simulink model "Practica1a__SemModSimulSist_Simulink"  (R2025b)
settings: Solver=VariableStepAuto  StartTime=0.0  StopTime=10.0  RelTol=1e-3
PreLoadFcn:
  | Ip = 0.0079;
  | Mc = 0.7031;
  | Lp = 0.3302;
  | Mp = 0.23;
  | Fc = 0;
  | Beq = 4.3;
  | g = 9.81;
  | Bp = 0.0024;
  | 
  | A = (Ip + Mp*(Lp^2))*Fc;
  | B = (Mp^2)*(Lp^2)*g;
  | C = (Ip + Mp*(Lp^2))*Beq;
  | D = Ip*Mp*Lp + (Mp^2)*(Lp^3); % Se cambio signo
  | E = Mp*Lp*Bp;
  | F = (Mc + Mp)*Mp*g*Lp;
  | G = (Mc + Mp)*Bp;
  | H = Fc*Mp*Lp;
  | K = (Mp^2)*(Lp^2);
  | M = Beq*Mp*Lp;
  | N = (Mc + Mp)*Ip + Mc*Mp*(Lp^2);
  | P = (Mp^2)*(Lp^2);
InitFcn:
  | Ip = 0.0079;
  | Mc = 0.7031;
  | Lp = 0.3302;
  | Mp = 0.23;
  | Fc = 0;
  | Beq = 4.3;
  | g = 9.81;
  | Bp = 0.0024;
  | 
  | 
  | A = (Ip + Mp*(Lp^2))*Fc;
  | 
  | B = (Mp^2)*(Lp^2)*g;
  | 
  | C = (Ip + Mp*(Lp^2))*Beq;
  | 
  | D = Ip*Mp*Lp + (Mp^2)*(Lp^3); % Se cambio signo
  | 
  | E = Mp*Lp*Bp;
  | 
  | F = (Mc + Mp)*Mp*g*Lp;
  | 
  | G = (Mc + Mp)*Bp;
  | 
  | H = Fc*Mp*Lp;
  | 
  | K = (Mp^2)*(Lp^2);
  | 
  | M = Beq*Mp*Lp;
  | 
  | N = (Mc + Mp)*Ip + Mc*Mp*(Lp^2);
  | 
  | P = (Mp^2)*(Lp^2);
undefined symbols (not defined in the file): magnitude
settings Model: Creator=jlsot  LastModifiedBy=jlsot

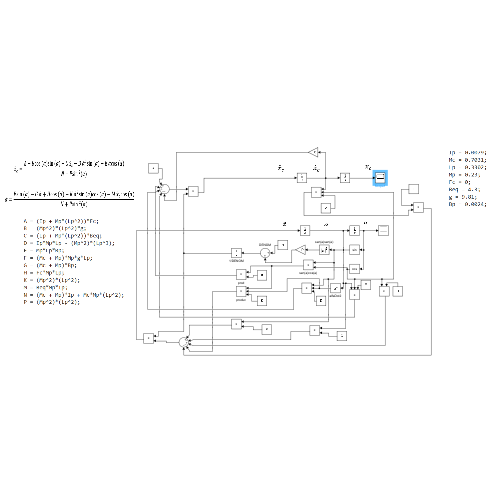
[thumbnail: Simulink's stored preview of the top-level diagram]
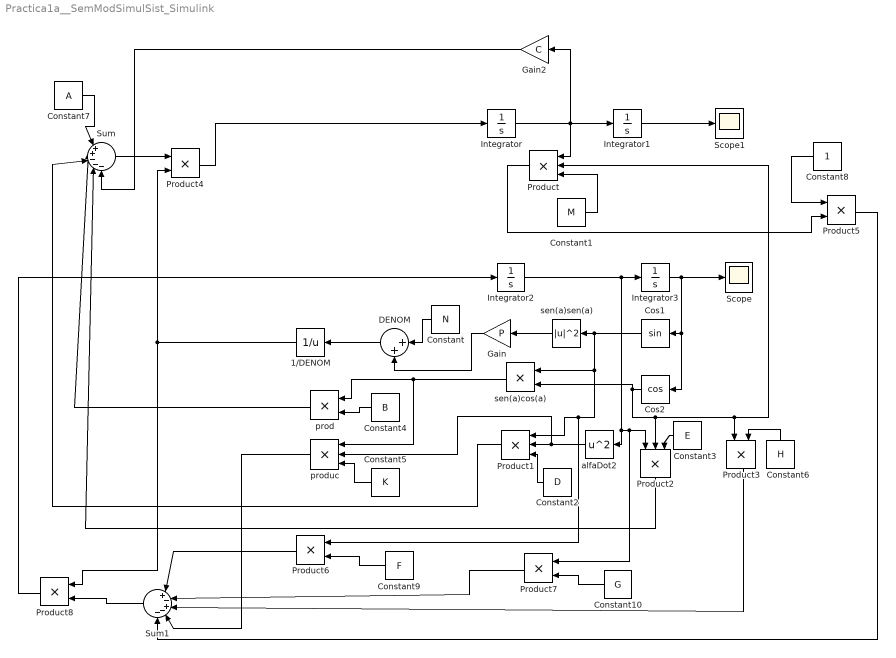
== system Practica1a__SemModSimulSist_Simulink ==
  1/DENOM : Math  Operator=reciprocal  SignedPower=on
  Constant : Constant  Value=N
  Constant1 : Constant  Value=M
  Constant10 : Constant  Value=G
  Constant2 : Constant  Value=D
  Constant3 : Constant  Value=E
  Constant4 : Constant  Value=B
  Constant5 : Constant  Value=K
  Constant6 : Constant  Value=H
  Constant7 : Constant  Value=A
  Constant8 : Constant
  Constant9 : Constant  Value=F
  Cos1 : Trigonometry
  Cos2 : Trigonometry  Operator=cos
  DENOM : Sum  Inputs=|++
  Gain : Gain  Gain=P
  Gain2 : Gain  Gain=C
  Integrator : Integrator
  Integrator1 : Integrator
  Integrator2 : Integrator
  Integrator3 : Integrator  InitialCondition=deg2rad(1)
  Product : Product  Inputs=3
  Product1 : Product  Inputs=3
  Product2 : Product  Inputs=3
  Product{3..8} (6 alike) : Product
  Scope : Scope
      settings: ActiveDisplayYMinimum=-0.63347576854008769  ActiveDisplayYMaximum=5.8758148420602225
  Scope1 : Scope
      settings: ActiveDisplayYMinimum=-0.11884151236554921  ActiveDisplayYMaximum=0.10920444319459102
  Sum : Sum  Inputs=|++---
  Sum1 : Sum  Inputs=|+-+--
  alfaDot2 : Math  Operator=square
  prod : Product
  produc : Product  Inputs=3
  sen(a)cos(a) : Product
  sen(a)sen(a) : Math  Operator=magnitude^2
  wires:
  Integrator/1 -> Gain2/1, Product/1, Integrator1/1
  Integrator2/1 -> Product7/1, Product2/1, alfaDot2/1, Integrator3/1
  sen(a)sen(a)/1 -> Gain/1
  Integrator3/1 -> Cos1/1, Cos2/1, Scope/1
  Cos1/1 -> sen(a)cos(a)/1, Product6/1, Product1/1, sen(a)sen(a)/1
  Integrator1/1 -> Scope1/1
  Cos2/1 -> sen(a)cos(a)/2, Product2/2, Product3/1, Product/2
  Constant/1 -> DENOM/1
  Gain/1 -> DENOM/2
  DENOM/1 -> 1/DENOM/1
  Constant1/1 -> Product/3
  Constant2/1 -> Product1/3
  Constant3/1 -> Product2/3
  sen(a)cos(a)/1 -> produc/1, prod/1
  Constant4/1 -> prod/2
  alfaDot2/1 -> produc/2, Product1/2
  Constant5/1 -> produc/3
  Constant6/1 -> Product3/2
  Constant7/1 -> Sum/1
  prod/1 -> Sum/2
  Gain2/1 -> Sum/5
  Product1/1 -> Sum/3
  Product2/1 -> Sum/4
  Sum/1 -> Product4/1
  1/DENOM/1 -> Product8/1, Product4/2
  Product4/1 -> Integrator/1
  Constant8/1 -> Product5/1
  Product/1 -> Product5/2
  Product5/1 -> Sum1/5
  produc/1 -> Sum1/4
  Product3/1 -> Sum1/3
  Constant9/1 -> Product6/2
  Product6/1 -> Sum1/1
  Constant10/1 -> Product7/2
  Product7/1 -> Sum1/2
  Sum1/1 -> Product8/2
  Product8/1 -> Integrator2/1
